simulink model "model"  (R2016a)
(part 2 of 2)

  T_242384114__POSTE_ZARZIS/RConn1 -- L_242384114/LConn1
  T_242384114__POSTE_ZARZIS/RConn2 -- L_242384114/LConn2
  L_242384114/LConn3 -- T_242384114__POSTE_ZARZIS/RConn3 -- bus67/LConn1
  T_178328237__POSTE_SIDI_MANSOUR/RConn1 -- L_178328237/LConn1
  T_178328237__POSTE_SIDI_MANSOUR/RConn2 -- L_178328237/LConn2
  L_178328237/LConn3 -- T_178328237__POSTE_SIDI_MANSOUR/RConn3 -- bus68/LConn1
  T_111375420__POSTE_SOUSSE/RConn1 -- L_111375420/LConn1
  T_111375420__POSTE_SOUSSE/RConn2 -- L_111375420/LConn2
  L_111375420/LConn3 -- T_111375420__POSTE_SOUSSE/RConn3 -- bus69/LConn1
  T_224416644__POSTE_OUESLATIA/RConn1 -- L_224416644/LConn1
  T_224416644__POSTE_OUESLATIA/RConn2 -- L_224416644/LConn2
  L_224416644/LConn3 -- T_224416644__POSTE_OUESLATIA/RConn3 -- bus70/LConn1
  T_224417135__POSTE_HAJEB_LAYOUN/RConn1 -- L_224417135/LConn1
  T_224417135__POSTE_HAJEB_LAYOUN/RConn2 -- L_224417135/LConn2
  L_224417135/LConn3 -- T_224417135__POSTE_HAJEB_LAYOUN/RConn3 -- bus71/LConn1
  T_173531194__POSTE_BIR_MCHARGA/RConn1 -- L_173531194/LConn1
  T_173531194__POSTE_BIR_MCHARGA/RConn2 -- L_173531194/LConn2
  L_173531194/LConn3 -- T_173531194__POSTE_BIR_MCHARGA/RConn3 -- bus72/LConn1
  T_129996167__/RConn1 -- L_129996167/LConn1
  T_129996167__/RConn2 -- L_129996167/LConn2
  L_129996167/LConn3 -- T_129996167__/RConn3 -- bus73/LConn1
  T_129996179__POSTE_MATEUR/RConn1 -- L_129996179/LConn1
  T_129996179__POSTE_MATEUR/RConn2 -- L_129996179/LConn2
  L_129996179/LConn3 -- T_129996179__POSTE_MATEUR/RConn3 -- bus74/LConn1
  T_101404944__POSTE_225_90_MNIHLA_1/RConn1 -- L_101404944/LConn1
  T_101404944__POSTE_225_90_MNIHLA_1/RConn2 -- L_101404944/LConn2
  L_101404944/LConn3 -- T_101404944__POSTE_225_90_MNIHLA_1/RConn3 -- bus75/LConn1
  T_125504235_225000_POSTE_NAASEN/RConn1 -- L_125504235/LConn1
  T_125504235_225000_POSTE_NAASEN/RConn2 -- L_125504235/LConn2
  L_125504235/LConn3 -- T_125504235_225000_POSTE_NAASEN/RConn3 -- bus76/LConn1
  T_179549833__POSTE_TAJEROUINE_225_KV/RConn1 -- L_179549833/LConn1
  T_179549833__POSTE_TAJEROUINE_225_KV/RConn2 -- L_179549833/LConn2
  L_179549833/LConn3 -- T_179549833__POSTE_TAJEROUINE_225_KV/RConn3 -- bus77/LConn1
  T_173534564__POSTE_JENDOUBA/RConn1 -- L_173534564/LConn1
  T_173534564__POSTE_JENDOUBA/RConn2 -- L_173534564/LConn2
  L_173534564/LConn3 -- T_173534564__POSTE_JENDOUBA/RConn3 -- bus78/LConn1
  T_178494278__POSTE_MENZEL_JEMIL/RConn1 -- L_178494278/LConn1
  T_178494278__POSTE_MENZEL_JEMIL/RConn2 -- L_178494278/LConn2
  L_178494278/LConn3 -- T_178494278__POSTE_MENZEL_JEMIL/RConn3 -- bus79/LConn1
  T_93263381__POSTE_RADES/RConn1 -- L_93263381/LConn1
  T_93263381__POSTE_RADES/RConn2 -- L_93263381/LConn2
  L_93263381/LConn3 -- T_93263381__POSTE_RADES/RConn3 -- bus80/LConn1
  T_189193646__POSTE_BOUCHEMMA/RConn1 -- L_189193646/LConn1
  T_189193646__POSTE_BOUCHEMMA/RConn2 -- L_189193646/LConn2
  L_189193646/LConn3 -- T_189193646__POSTE_BOUCHEMMA/RConn3 -- bus81/LConn1
  T_180611326__POSTE_MEDENINE/RConn1 -- L_180611326/LConn1
  T_180611326__POSTE_MEDENINE/RConn2 -- L_180611326/LConn2
  L_180611326/LConn3 -- T_180611326__POSTE_MEDENINE/RConn3 -- bus82/LConn1
  T_180615776__POSTE_TATAOUINE/RConn1 -- L_180615776/LConn1
  T_180615776__POSTE_TATAOUINE/RConn2 -- L_180615776/LConn2
  L_180615776/LConn3 -- T_180615776__POSTE_TATAOUINE/RConn3 -- bus83/LConn1
  T_242398869__POSTE_KAIROUAN/RConn1 -- L_242398869/LConn1
  T_242398869__POSTE_KAIROUAN/RConn2 -- L_242398869/LConn2
  L_242398869/LConn3 -- T_242398869__POSTE_KAIROUAN/RConn3 -- bus84/LConn1
  T_226848748__/RConn1 -- L_226848748/LConn1
  T_226848748__/RConn2 -- L_226848748/LConn2
  L_226848748/LConn3 -- T_226848748__/RConn3 -- bus85/LConn1
